simulink model "МатЛаба2"  (Simulink 4.00)
settings: Solver=ode45  StartTime=0.0  StopTime=50  RelTol=1e-3
libraries: cstblocks x2
settings Model: LastModifiedBy=Õîçÿèí

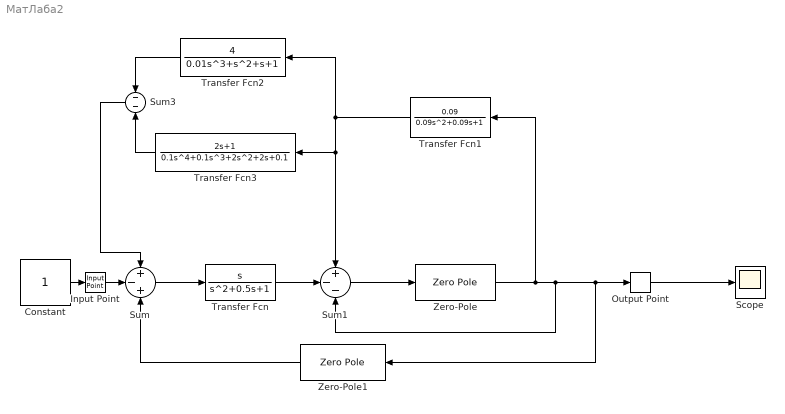
== system МатЛаба2 ==
  Constant : Constant  Value=1
  Input Point : cstblocks/Input Point
  Output Point : cstblocks/Output Point
  Scope : Scope
      settings: TimeRange=20  YMin=-300  YMax=50  SaveToWorkspace=off  SaveName=ScopeData  LimitDataPoints=on  MaxDataPoints=5000
  Sum : Sum  Inputs=+-+  SaturateOnIntegerOverflow=on
  Sum1 : Sum  Inputs=+--  SaturateOnIntegerOverflow=on
  Sum3 : Sum  Orientation=left  Inputs=--  SaturateOnIntegerOverflow=on
  Transfer Fcn : TransferFcn  Numerator=[1 0]  Denominator=[1 0.5 1]  AbsoluteTolerance=auto  Realization=auto
  Transfer Fcn1 : TransferFcn  Orientation=left  Numerator=[0.09]  Denominator=[0.09 0.09 1]  AbsoluteTolerance=auto  Realization=auto
  Transfer Fcn2 : TransferFcn  Orientation=left  Numerator=[4]  Denominator=[0.01 1 1 1]  AbsoluteTolerance=auto  Realization=auto
  Transfer Fcn3 : TransferFcn  Orientation=left  Numerator=[2 1]  Denominator=[0.1 0.1 2 2 0.1]  AbsoluteTolerance=auto  Realization=auto
  Zero-Pole : ZeroPole  Zeros=[0]  Poles=[-0.04 -0.04]  Gain=[1]  AbsoluteTolerance=auto
  Zero-Pole1 : ZeroPole  Orientation=left  Zeros=[0]  Poles=[-0.09 0.09]  Gain=[1]  AbsoluteTolerance=auto
  wires:
  Sum1/1 -> Zero-Pole/1
  Sum/1 -> Transfer Fcn/1
  Transfer Fcn1/1 -> Transfer Fcn2/1, Sum1/1, Transfer Fcn3/1
  Transfer Fcn/1 -> Sum1/2
  Transfer Fcn2/1 -> Sum3/1
  Transfer Fcn3/1 -> Sum3/2
  Sum3/1 -> Sum/1
  Zero-Pole/1 -> Transfer Fcn1/1, Sum1/3, Zero-Pole1/1, Output Point/1
  Zero-Pole1/1 -> Sum/3
  Constant/1 -> Input Point/1
  Input Point/1 -> Sum/2
  Output Point/1 -> Scope/1
